simulink model "sinusoidtracking"  (R2023a)
settings: Solver=VariableStepAuto  StartTime=0.0  StopTime=10.0  RelTol=1e-3
values from neighbouring files (symbols this model uses):
  C = [0 1 0 0 0]    [obsv_ctrb.m]    (also in reduced_order.m = [0 1 0 0]; testobsv.m = [1 0 0 0 0])
  K_sin_int = K_sin(1)    [sinusoid.m]
  K_sin_x = K_sin(2:5)    [sinusoid.m]
  x1_bar = deg2rad(31.78)    [reduced_order.m]
  x2_bar = deg2rad(30)    [reduced_order.m]
undefined symbols (not defined in the file or in its folder): g, I_noload, init, K_m, l, m, R
settings Model: Creator=yunzh  LastModifiedBy=yunzh

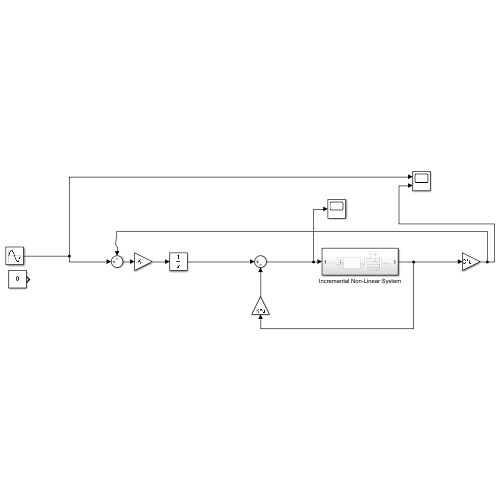
[thumbnail: Simulink's stored preview of the top-level diagram]
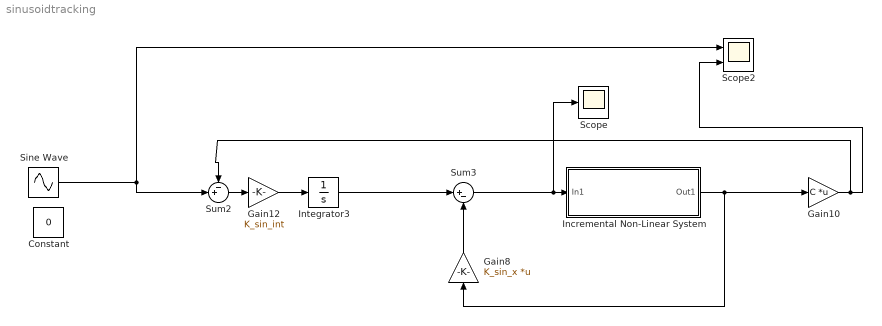
== system sinusoidtracking ==
  Constant : Constant  Value=0
  Gain10 : Gain  Gain=C  Multiplication=Matrix(K*u)
  Gain12 : Gain  Gain=K_sin_int
  Gain8 : Gain  Gain=K_sin_x  Multiplication=Matrix(K*u)
  Incremental Non-Linear System : Subsystem
  Integrator3 : Integrator
  Scope : Scope
  Scope2 : Scope  NumInputPorts=2
  Sine Wave : Sin  Amplitude=deg2rad(25)  Bias=deg2rad(-5)  Frequency=2*pi/4  SampleTime=0
  Sum2 : Sum  Inputs=-+|
  Sum3 : Sum  Inputs=|+-
  wires:
  Sum3/1 -> Scope/1, Incremental Non-Linear System/1(In1)
  Incremental Non-Linear System/1(Out1) -> Gain8/1, Gain10/1
  Sine Wave/1 -> Sum2/2, Scope2/1
  Gain8/1 -> Sum3/2
  Gain12/1 -> Integrator3/1
  Gain10/1 -> Sum2/1, Scope2/2
  Sum2/1 -> Gain12/1
  Integrator3/1 -> Sum3/1

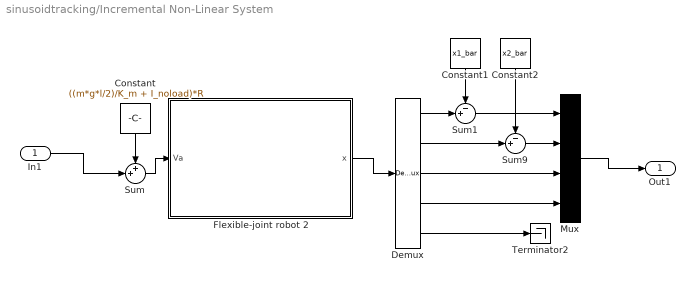
== system sinusoidtracking/Incremental Non-Linear System ==
  In1 : Inport
  Constant : Constant  Value=((m*g*l/2)/K_m + I_noload)*R
  Constant1 : Constant  Value=x1_bar
  Constant2 : Constant  Value=x2_bar
  Demux : Demux  Outputs=5
  Flexible-joint robot 2 : Subsystem
      mask Display: image('$imagefile'); % Use "Edit Image" on toolstrip to change.
  Mux : Mux
  Sum : Sum  Inputs=++|
  Sum1 : Sum  Inputs=-+|
  Sum9 : Sum  Inputs=-+|
  Terminator2 : Terminator
  Out1 : Outport
  wires:
  Flexible-joint robot 2/1(x) -> Demux/1
  Demux/1 -> Sum1/2
  Demux/2 -> Sum9/2
  Demux/5 -> Terminator2/1
  Sum/1 -> Flexible-joint robot 2/1(Va)
  Constant1/1 -> Sum1/1
  Sum9/1 -> Mux/2
  Constant2/1 -> Sum9/1
  Sum1/1 -> Mux/1
  Demux/4 -> Mux/4
  Demux/3 -> Mux/3
  Constant/1 -> Sum/1
  In1/1 -> Sum/2
  Mux/1 -> Out1/1

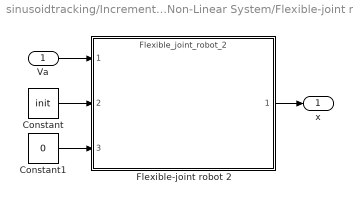
== system sinusoidtracking/Incremental Non-Linear System/Flexible-joint robot 2 ==
  Va : Inport
  Constant : Constant  Value=init
  Constant1 : Constant  Value=0
  Flexible-joint robot 2 : ModelReference  ModelNameDialog=Flexible_joint_robot_2  ModelReferenceVersion=1.65  CopyOfModelProtected=on
  x : Outport
  wires:
  Va/1 -> Flexible-joint robot 2/1
  Constant1/1 -> Flexible-joint robot 2/3
  Constant/1 -> Flexible-joint robot 2/2
  Flexible-joint robot 2/1 -> x/1
